simulink model "ASW_SigIn"  (R2023a)
settings: configuration reference "cfg_FastTaskCodeGeneration_v01" (kept outside this file)
undefined symbols (not defined in the file): Cdbl_tiMedTaskSmpTi, Cdbl_tiSlwTaskSmpTi
settings Model: DataDictionary=dd_foc_dictionary.sldd  EnableAccessToBaseWorkspace=off  Creator=WFYXQ  LastModifiedBy=xiaoqiang.yuan
settings ConfigSetRef: SourceName=cfg_FastTaskCodeGeneration_v01

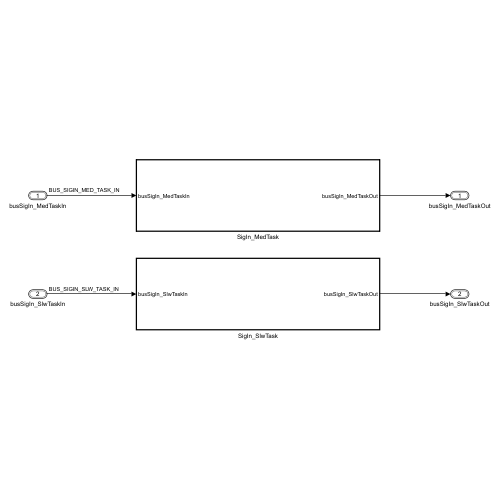
[thumbnail: Simulink's stored preview of the top-level diagram]
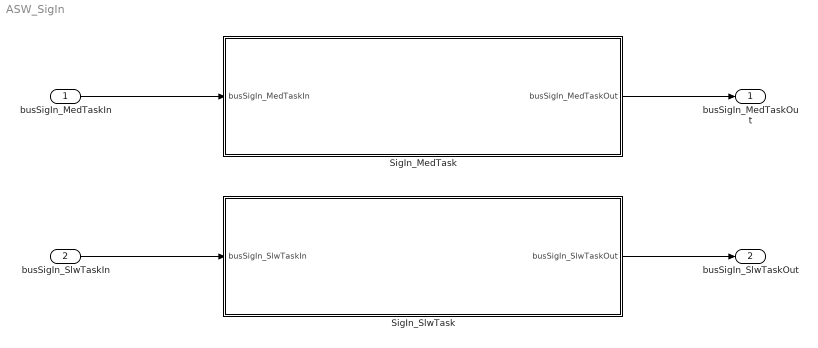
== system ASW_SigIn ==
  busSigIn_MedTaskIn : Inport  OutDataTypeStr=Bus: BUS_SIGIN_MED_TASK_IN  SampleTime=round(double(Cdbl_tiMedTaskSmpTi),6)  BusOutputAsStruct=on
  busSigIn_SlwTaskIn : Inport  Port=2  OutDataTypeStr=Bus: BUS_SIGIN_SLW_TASK_IN  SampleTime=round(double(Cdbl_tiSlwTaskSmpTi),4)  BusOutputAsStruct=on
  SigIn_MedTask : Subsystem  TreatAsAtomicUnit=on  RTWFcnName=SigIn_MedTask
      settings: RTWSystemCode=Nonreusable function  RTWFcnNameOpts=User specified
  SigIn_SlwTask : Subsystem  TreatAsAtomicUnit=on  RTWFcnName=SigIn_SlwTask
      settings: RTWSystemCode=Nonreusable function  RTWFcnNameOpts=User specified
  busSigIn_MedTaskOut : Outport  OutDataTypeStr=Bus: BUS_SIGIN_MED_TASK_OUT  SampleTime=round(double(Cdbl_tiMedTaskSmpTi),6)
  busSigIn_SlwTaskOut : Outport  Port=2  OutDataTypeStr=Bus: BUS_SIGIN_SLW_TASK_OUT  SampleTime=round(double(Cdbl_tiSlwTaskSmpTi),4)
  wires:
  busSigIn_MedTaskIn/1 -> SigIn_MedTask/1(busSigIn_MedTaskIn)
  SigIn_MedTask/1(busSigIn_MedTaskOut) -> busSigIn_MedTaskOut/1
  SigIn_SlwTask/1(busSigIn_SlwTaskOut) -> busSigIn_SlwTaskOut/1
  busSigIn_SlwTaskIn/1 -> SigIn_SlwTask/1(busSigIn_SlwTaskIn)

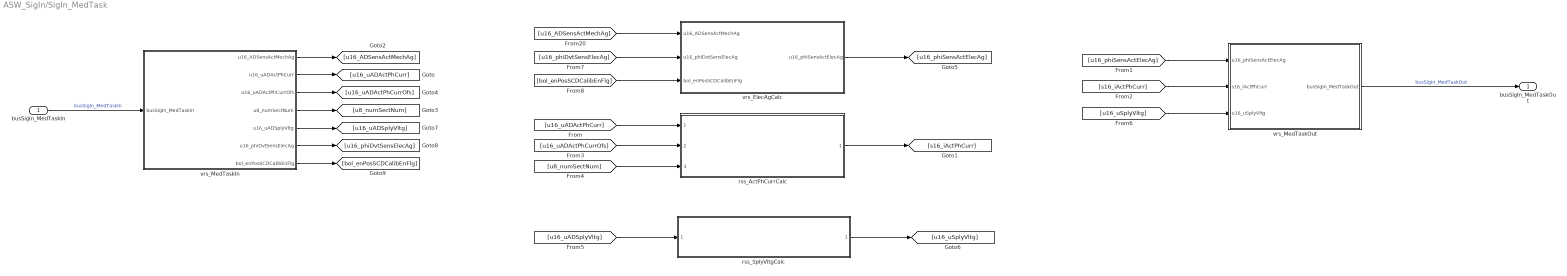
== system ASW_SigIn/SigIn_MedTask ==
  busSigIn_MedTaskIn : Inport
  rss_ActPhCurrCalc : Subsystem  ReferencedSubsystem=rss_ActPhCurrCalc
  rss_SplyVltgCalc : Subsystem  ReferencedSubsystem=rss_SplyVltgCalc
  vrs_ElecAgCalc : Subsystem  Variant=on  VariantControlMode=label  VariantControl=Choice  LabelModeActiveChoice=cstSensCtrlLbl
  vrs_MedTaskIn : Subsystem  Variant=on  VariantControlMode=label  VariantControl=cstSenlCtrlLbl  LabelModeActiveChoice=cstSensCtrlLbl
  vrs_MedTaskOut : Subsystem  Variant=on  VariantControlMode=label  VariantControl=Choice  LabelModeActiveChoice=cstSensCtrlLbl
  busSigIn_MedTaskOut : Outport
  wires:
  vrs_MedTaskOut/1(busSigIn_MedTaskOut) -> busSigIn_MedTaskOut/1  "busSigIn_MedTaskOut"
  [u16_phiSensActElecAg] -> vrs_MedTaskOut/1(u16_phiSensActElecAg)
  rss_ActPhCurrCalc/1 -> [s16_iActPhCurr]
  [u16_uADActPhCurr] -> rss_ActPhCurrCalc/1
  [s16_iActPhCurr] -> vrs_MedTaskOut/2(s16_iActPhCurr)
  [u16_uADActPhCurrOfs] -> rss_ActPhCurrCalc/2
  [u8_numSectNum] -> rss_ActPhCurrCalc/3
  [u16_ADSensActMechAg] -> vrs_ElecAgCalc/1(u16_ADSensActMechAg)
  vrs_ElecAgCalc/1(u16_phiSensActElecAg) -> [u16_phiSensActElecAg]
  busSigIn_MedTaskIn/1 -> vrs_MedTaskIn/1(busSigIn_MedTaskIn)  "busSigIn_MedTaskIn"
  vrs_MedTaskIn/1(u16_ADSensActMechAg) -> [u16_ADSensActMechAg]
  vrs_MedTaskIn/2(u16_uADActPhCurr) -> [u16_uADActPhCurr]
  vrs_MedTaskIn/3(u16_uADActPhCurrOfs) -> [u16_uADActPhCurrOfs]
  vrs_MedTaskIn/4(u8_numSectNum) -> [u8_numSectNum]
  [u16_uADSplyVltg] -> rss_SplyVltgCalc/1
  rss_SplyVltgCalc/1 -> [u16_uSplyVltg]
  vrs_MedTaskIn/5(u16_uADSplyVltg) -> [u16_uADSplyVltg]
  [u16_uSplyVltg] -> vrs_MedTaskOut/3(u16_uSplyVltg)
  [u16_phiDvtSensElecAg] -> vrs_ElecAgCalc/2(u16_phiDvtSensElecAg)
  [bol_enPosSCDCalibEnFlg] -> vrs_ElecAgCalc/3(bol_enPosSCDCalibEnFlg)
  vrs_MedTaskIn/6(u16_phiDvtSensElecAg) -> [u16_phiDvtSensElecAg]
  vrs_MedTaskIn/7(bol_enPosSCDCalibEnFlg) -> [bol_enPosSCDCalibEnFlg]

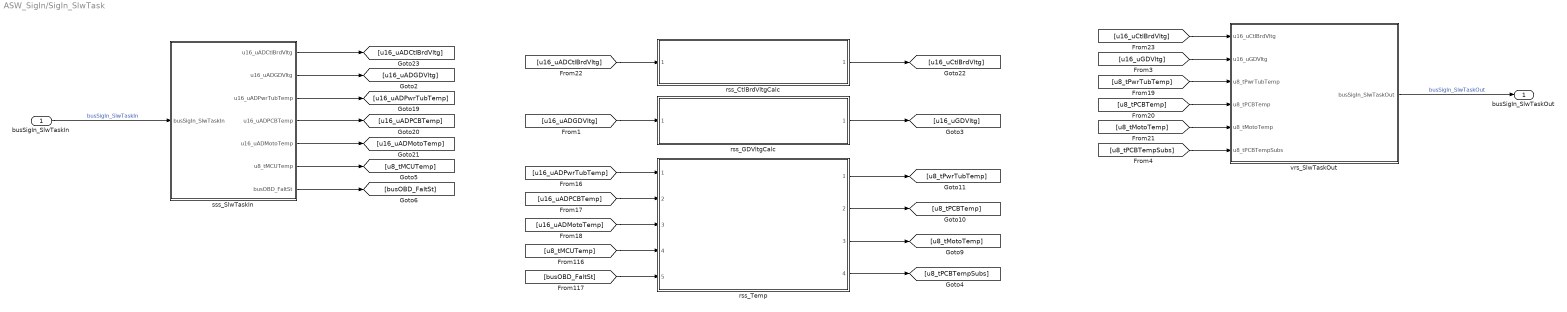
== system ASW_SigIn/SigIn_SlwTask ==
  busSigIn_SlwTaskIn : Inport
  rss_CtlBrdVltgCalc : Subsystem  ReferencedSubsystem=rss_CtlBrdVltgCalc
  rss_GDVltgCalc : Subsystem  ReferencedSubsystem=rss_GDVltgCalc
  rss_Temp : Subsystem  ReferencedSubsystem=rss_Temp
  sss_SlwTaskIn : Subsystem  VariantControl=cstSenlCtrlLbl
  vrs_SlwTaskOut : Subsystem  Variant=on  VariantControlMode=label  VariantControl=Choice  LabelModeActiveChoice=cstSenlCtrlLbl
  busSigIn_SlwTaskOut : Outport
  wires:
  busSigIn_SlwTaskIn/1 -> sss_SlwTaskIn/1(busSigIn_SlwTaskIn)  "busSigIn_SlwTaskIn"
  vrs_SlwTaskOut/1(busSigIn_SlwTaskOut) -> busSigIn_SlwTaskOut/1  "busSigIn_SlwTaskOut"
  [u16_uADPwrTubTemp] -> rss_Temp/1
  [u16_uADPCBTemp] -> rss_Temp/2
  [u16_uADMotoTemp] -> rss_Temp/3
  rss_Temp/1 -> [u8_tPwrTubTemp]
  rss_Temp/2 -> [u8_tPCBTemp]
  rss_Temp/3 -> [u8_tMotoTemp]
  [u8_tPwrTubTemp] -> vrs_SlwTaskOut/3(u8_tPwrTubTemp)
  [u8_tPCBTemp] -> vrs_SlwTaskOut/4(u8_tPCBTemp)
  [u8_tMotoTemp] -> vrs_SlwTaskOut/5(u8_tMotoTemp)
  sss_SlwTaskIn/3(u16_uADPwrTubTemp) -> [u16_uADPwrTubTemp]
  sss_SlwTaskIn/4(u16_uADPCBTemp) -> [u16_uADPCBTemp]
  sss_SlwTaskIn/5(u16_uADMotoTemp) -> [u16_uADMotoTemp]
  rss_CtlBrdVltgCalc/1 -> [u16_uCtlBrdVltg]
  [u16_uADCtlBrdVltg] -> rss_CtlBrdVltgCalc/1
  [u16_uCtlBrdVltg] -> vrs_SlwTaskOut/1(u16_uCtlBrdVltg)
  sss_SlwTaskIn/1(u16_uADCtlBrdVltg) -> [u16_uADCtlBrdVltg]
  sss_SlwTaskIn/2(u16_uADGDVltg) -> [u16_uADGDVltg]
  [u16_uADGDVltg] -> rss_GDVltgCalc/1
  rss_GDVltgCalc/1 -> [u16_uGDVltg]
  [u16_uGDVltg] -> vrs_SlwTaskOut/2(u16_uGDVltg)
  [u8_tMCUTemp] -> rss_Temp/4
  [busOBD_FaltSt] -> rss_Temp/5
  rss_Temp/4 -> [u8_tPCBTempSubs]
  sss_SlwTaskIn/6(u8_tMCUTemp) -> [u8_tMCUTemp]
  sss_SlwTaskIn/7(busOBD_FaltSt) -> [busOBD_FaltSt]
  [u8_tPCBTempSubs] -> vrs_SlwTaskOut/6(u8_tPCBTempSubs)

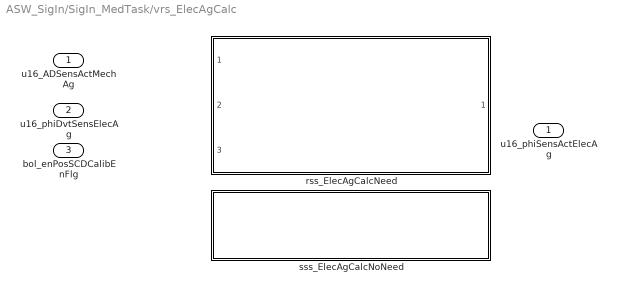
== system ASW_SigIn/SigIn_MedTask/vrs_ElecAgCalc ==
  u16_ADSensActMechAg : Inport
  u16_phiDvtSensElecAg : Inport  Port=2
  bol_enPosSCDCalibEnFlg : Inport  Port=3
  rss_ElecAgCalcNeed : Subsystem  VariantControl=cstSensCtrlLbl  ReferencedSubsystem=rss_ElecAgCalcNeed
  sss_ElecAgCalcNoNeed : Subsystem  VariantControl=cstSenlCtrlLbl
  u16_phiSensActElecAg : Outport

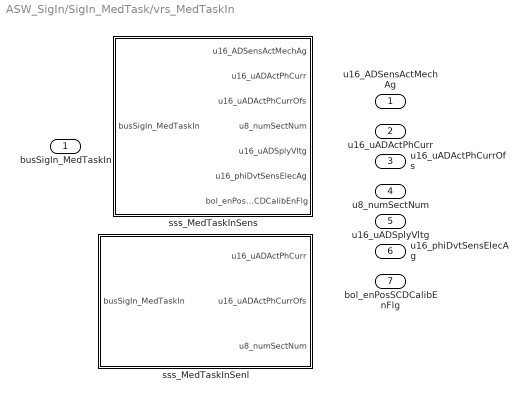
== system ASW_SigIn/SigIn_MedTask/vrs_MedTaskIn ==
  busSigIn_MedTaskIn : Inport
  sss_MedTaskInSenl : Subsystem  VariantControl=cstSenlCtrlLbl
  sss_MedTaskInSens : Subsystem  VariantControl=cstSensCtrlLbl
  u16_ADSensActMechAg : Outport
  u16_uADActPhCurr : Outport  Port=2
  u16_uADActPhCurrOfs : Outport  Port=3
  u8_numSectNum : Outport  Port=4
  u16_uADSplyVltg : Outport  Port=5
  u16_phiDvtSensElecAg : Outport  Port=6
  bol_enPosSCDCalibEnFlg : Outport  Port=7

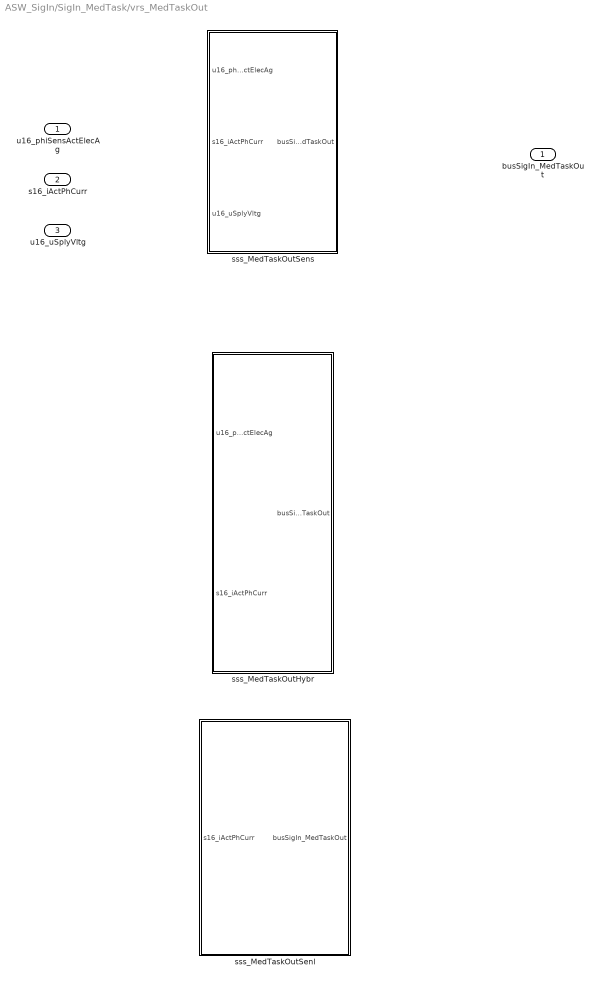
== system ASW_SigIn/SigIn_MedTask/vrs_MedTaskOut ==
  u16_phiSensActElecAg : Inport
  s16_iActPhCurr : Inport  Port=2
  u16_uSplyVltg : Inport  Port=3
  sss_MedTaskOutHybr : Subsystem  VariantControl=cstHybrCtrlLbl
  sss_MedTaskOutSenl : Subsystem  VariantControl=cstSenlCtrlLbl
  sss_MedTaskOutSens : Subsystem  VariantControl=cstSensCtrlLbl
  busSigIn_MedTaskOut : Outport

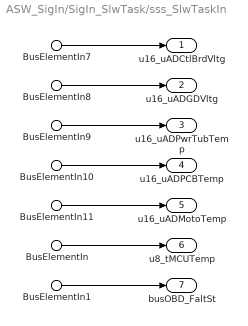
== system ASW_SigIn/SigIn_SlwTask/sss_SlwTaskIn ==
  BusElementIn7 : Inport  PortName=busSigIn_SlwTaskIn  Element=u16_uADCtlBrdVltg
  BusElementIn8 : Inport  PortName=busSigIn_SlwTaskIn  Element=u16_uADGDVltg
  BusElementIn9 : Inport  PortName=busSigIn_SlwTaskIn  Element=u16_uADPwrTubTemp
  BusElementIn10 : Inport  PortName=busSigIn_SlwTaskIn  Element=u16_uADPCBTemp
  BusElementIn11 : Inport  PortName=busSigIn_SlwTaskIn  Element=u16_uADMotoTemp
  BusElementIn : Inport  PortName=busSigIn_SlwTaskIn  Element=u8_tMCUTemp
  BusElementIn1 : Inport  PortName=busSigIn_SlwTaskIn  Element=busOBD_FaltSt
  u16_uADCtlBrdVltg : Outport
  u16_uADGDVltg : Outport  Port=2
  u16_uADPwrTubTemp : Outport  Port=3
  u16_uADPCBTemp : Outport  Port=4
  u16_uADMotoTemp : Outport  Port=5
  u8_tMCUTemp : Outport  Port=6
  busOBD_FaltSt : Outport  Port=7
  wires:
  BusElementIn9/1 -> u16_uADPwrTubTemp/1
  BusElementIn10/1 -> u16_uADPCBTemp/1
  BusElementIn11/1 -> u16_uADMotoTemp/1
  BusElementIn7/1 -> u16_uADCtlBrdVltg/1
  BusElementIn8/1 -> u16_uADGDVltg/1
  BusElementIn/1 -> u8_tMCUTemp/1
  BusElementIn1/1 -> busOBD_FaltSt/1

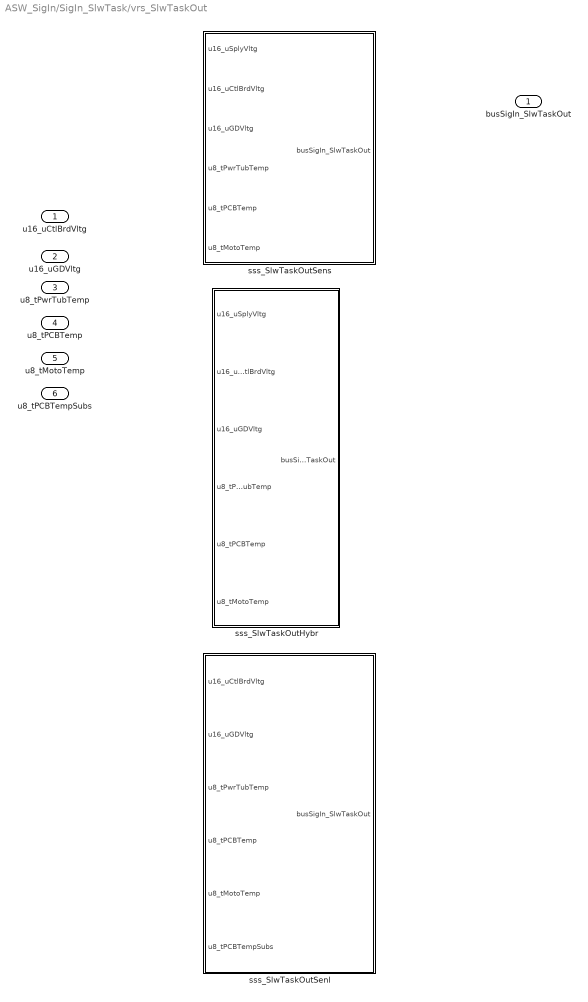
== system ASW_SigIn/SigIn_SlwTask/vrs_SlwTaskOut ==
  u16_uCtlBrdVltg : Inport
  u16_uGDVltg : Inport  Port=2
  u8_tPwrTubTemp : Inport  Port=3
  u8_tPCBTemp : Inport  Port=4
  u8_tMotoTemp : Inport  Port=5
  u8_tPCBTempSubs : Inport  Port=6
  sss_SlwTaskOutHybr : Subsystem  VariantControl=cstHybrCtrlLbl
  sss_SlwTaskOutSenl : Subsystem  VariantControl=cstSenlCtrlLbl
  sss_SlwTaskOutSens : Subsystem  VariantControl=cstSensCtrlLbl
  busSigIn_SlwTaskOut : Outport

== system ASW_SigIn/SigIn_MedTask/vrs_ElecAgCalc/sss_ElecAgCalcNoNeed ==

== system ASW_SigIn/SigIn_MedTask/vrs_MedTaskIn/sss_MedTaskInSenl ==
  BusElementIn7 : Inport  PortName=busSigIn_MedTaskIn  Element=u8_numSectNum
  BusElementIn : Inport  PortName=busSigIn_MedTaskIn  Element=s16_uADActPhCurr
  BusElementIn1 : Inport  PortName=busSigIn_MedTaskIn  Element=s16_uADActPhCurrOfs
  u16_uADActPhCurr : Outport
  u16_uADActPhCurrOfs : Outport  Port=2
  u8_numSectNum : Outport  Port=3
  wires:
  BusElementIn/1 -> u16_uADActPhCurr/1
  BusElementIn1/1 -> u16_uADActPhCurrOfs/1
  BusElementIn7/1 -> u8_numSectNum/1

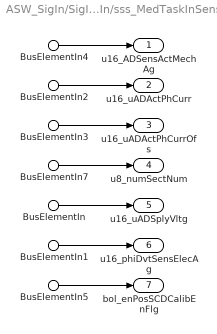
== system ASW_SigIn/SigIn_MedTask/vrs_MedTaskIn/sss_MedTaskInSens ==
  BusElementIn4 : Inport  PortName=busSigIn_MedTaskIn  Element=u16_ADSensActMechAg
  BusElementIn7 : Inport  PortName=busSigIn_MedTaskIn  Element=u8_numSectNum
  BusElementIn2 : Inport  PortName=busSigIn_MedTaskIn  Element=u16_uADActPhCurr
  BusElementIn3 : Inport  PortName=busSigIn_MedTaskIn  Element=u16_uADActPhCurrOfs
  BusElementIn : Inport  PortName=busSigIn_MedTaskIn  Element=u16_uADSplyVltg
  BusElementIn1 : Inport  PortName=busSigIn_MedTaskIn  Element=u16_phiDvtSensElecAg
  BusElementIn5 : Inport  PortName=busSigIn_MedTaskIn  Element=bol_enPosSCDCalibEnFlg
  u16_ADSensActMechAg : Outport
  u16_uADActPhCurr : Outport  Port=2
  u16_uADActPhCurrOfs : Outport  Port=3
  u8_numSectNum : Outport  Port=4
  u16_uADSplyVltg : Outport  Port=5
  u16_phiDvtSensElecAg : Outport  Port=6
  bol_enPosSCDCalibEnFlg : Outport  Port=7
  wires:
  BusElementIn4/1 -> u16_ADSensActMechAg/1
  BusElementIn2/1 -> u16_uADActPhCurr/1
  BusElementIn3/1 -> u16_uADActPhCurrOfs/1
  BusElementIn7/1 -> u8_numSectNum/1
  BusElementIn/1 -> u16_uADSplyVltg/1
  BusElementIn1/1 -> u16_phiDvtSensElecAg/1
  BusElementIn5/1 -> bol_enPosSCDCalibEnFlg/1

== system ASW_SigIn/SigIn_MedTask/vrs_MedTaskOut/sss_MedTaskOutHybr ==
  u16_phiSensActElecAg : Inport
  s16_iActPhCurr : Inport  Port=2
  Bus Creator1 : BusCreator  Inputs=2  OutDataTypeStr=Bus: BUS_SIGIN_MED_TASK_OUT  NonVirtualBus=on
      settings: InheritFromInputs=off
  busSigIn_MedTaskOut : Outport
  wires:
  Bus Creator1/1 -> busSigIn_MedTaskOut/1
  s16_iActPhCurr/1 -> Bus Creator1/2
  u16_phiSensActElecAg/1 -> Bus Creator1/1

== system ASW_SigIn/SigIn_MedTask/vrs_MedTaskOut/sss_MedTaskOutSenl ==
  s16_iActPhCurr : Inport
  Bus Creator1 : BusCreator  Inputs=1  OutDataTypeStr=Bus: BUS_SIGIN_MED_TASK_OUT  NonVirtualBus=on
      settings: InheritFromInputs=off
  busSigIn_MedTaskOut : Outport
  wires:
  Bus Creator1/1 -> busSigIn_MedTaskOut/1
  s16_iActPhCurr/1 -> Bus Creator1/1

== system ASW_SigIn/SigIn_MedTask/vrs_MedTaskOut/sss_MedTaskOutSens ==
  u16_phiSensActElecAg : Inport
  s16_iActPhCurr : Inport  Port=2
  u16_uSplyVltg : Inport  Port=3
  Bus Creator1 : BusCreator  Inputs=3  OutDataTypeStr=Bus: BUS_SIGIN_MED_TASK_OUT  NonVirtualBus=on
      settings: InheritFromInputs=off
  busSigIn_MedTaskOut : Outport
  wires:
  Bus Creator1/1 -> busSigIn_MedTaskOut/1
  u16_phiSensActElecAg/1 -> Bus Creator1/1
  s16_iActPhCurr/1 -> Bus Creator1/2
  u16_uSplyVltg/1 -> Bus Creator1/3

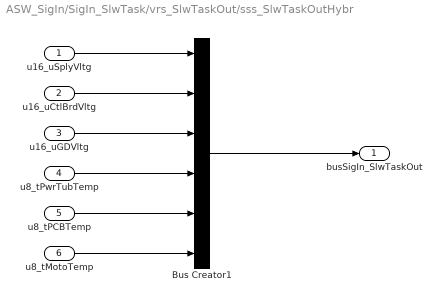
== system ASW_SigIn/SigIn_SlwTask/vrs_SlwTaskOut/sss_SlwTaskOutHybr ==
  u16_uSplyVltg : Inport
  u16_uCtlBrdVltg : Inport  Port=2
  u16_uGDVltg : Inport  Port=3
  u8_tPwrTubTemp : Inport  Port=4
  u8_tPCBTemp : Inport  Port=5
  u8_tMotoTemp : Inport  Port=6
  Bus Creator1 : BusCreator  Inputs=6  OutDataTypeStr=Bus: BUS_SIGIN_SLW_TASK_OUT  NonVirtualBus=on
      settings: InheritFromInputs=off
  busSigIn_SlwTaskOut : Outport
  wires:
  u8_tMotoTemp/1 -> Bus Creator1/6
  Bus Creator1/1 -> busSigIn_SlwTaskOut/1
  u16_uGDVltg/1 -> Bus Creator1/3
  u8_tPCBTemp/1 -> Bus Creator1/5
  u16_uCtlBrdVltg/1 -> Bus Creator1/2
  u8_tPwrTubTemp/1 -> Bus Creator1/4
  u16_uSplyVltg/1 -> Bus Creator1/1

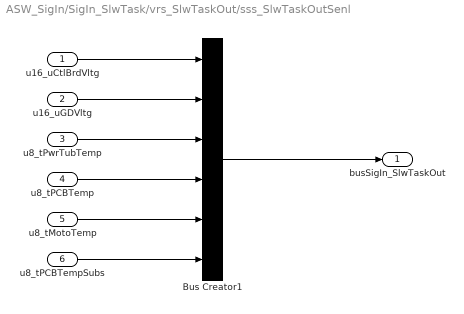
== system ASW_SigIn/SigIn_SlwTask/vrs_SlwTaskOut/sss_SlwTaskOutSenl ==
  u16_uCtlBrdVltg : Inport
  u16_uGDVltg : Inport  Port=2
  u8_tPwrTubTemp : Inport  Port=3
  u8_tPCBTemp : Inport  Port=4
  u8_tMotoTemp : Inport  Port=5
  u8_tPCBTempSubs : Inport  Port=6
  Bus Creator1 : BusCreator  Inputs=6  OutDataTypeStr=Bus: BUS_SIGIN_SLW_TASK_OUT  NonVirtualBus=on
      settings: InheritFromInputs=off
  busSigIn_SlwTaskOut : Outport
  wires:
  Bus Creator1/1 -> busSigIn_SlwTaskOut/1
  u16_uCtlBrdVltg/1 -> Bus Creator1/1
  u16_uGDVltg/1 -> Bus Creator1/2
  u8_tPwrTubTemp/1 -> Bus Creator1/3
  u8_tPCBTemp/1 -> Bus Creator1/4
  u8_tMotoTemp/1 -> Bus Creator1/5
  u8_tPCBTempSubs/1 -> Bus Creator1/6

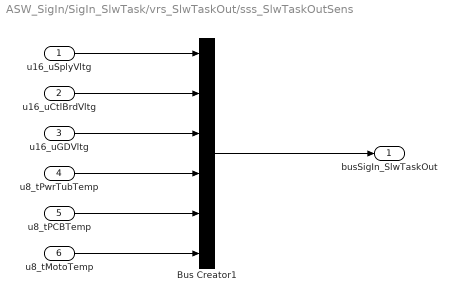
== system ASW_SigIn/SigIn_SlwTask/vrs_SlwTaskOut/sss_SlwTaskOutSens ==
  u16_uSplyVltg : Inport
  u16_uCtlBrdVltg : Inport  Port=2
  u16_uGDVltg : Inport  Port=3
  u8_tPwrTubTemp : Inport  Port=4
  u8_tPCBTemp : Inport  Port=5
  u8_tMotoTemp : Inport  Port=6
  Bus Creator1 : BusCreator  Inputs=6  OutDataTypeStr=Bus: BUS_SIGIN_SLW_TASK_OUT  NonVirtualBus=on
      settings: InheritFromInputs=off
  busSigIn_SlwTaskOut : Outport
  wires:
  Bus Creator1/1 -> busSigIn_SlwTaskOut/1
  u16_uSplyVltg/1 -> Bus Creator1/1
  u16_uCtlBrdVltg/1 -> Bus Creator1/2
  u8_tMotoTemp/1 -> Bus Creator1/6
  u8_tPCBTemp/1 -> Bus Creator1/5
  u8_tPwrTubTemp/1 -> Bus Creator1/4
  u16_uGDVltg/1 -> Bus Creator1/3
